simulink library "GenericINSLibrary"  (R2020b)
settings: Solver=VariableStepAuto  StartTime=0.0  StopTime=10.0  RelTol=1e-3
libraries: simulink x44
(part 2 of 6)

== system GenericINSLibrary/Empty Bus Sensor Fusion/GNSS4 ==
  Bus Creator : BusCreator  Inputs=1
  Bus Creator1 : BusCreator  Inputs=3
  Bus Creator2 : BusCreator  Inputs=3
  Bus Creator3 : BusCreator  Inputs=4
  Constant71 : Constant  Value=[0;0;0]  OutDataTypeStr=double
  Constant72 : Constant  OutDataTypeStr=double
  Constant73 : Constant  OutDataTypeStr=double
  Constant74 : Constant  OutDataTypeStr=double
  Constant{75..78} (4 alike) : Constant  Value=0  OutDataTypeStr=double
  Signal Specification : SignalSpecification  OutDataTypeStr=double  Unit=m  Dimensions=3
  Signal Specification{1..3,7} (4 alike) : SignalSpecification  OutDataTypeStr=double  Unit=m  Dimensions=1
  Signal Specification4 : SignalSpecification  OutDataTypeStr=double  Unit=s  Dimensions=1
  Signal Specification5 : SignalSpecification  OutDataTypeStr=double  Unit=rad  Dimensions=1
  Signal Specification6 : SignalSpecification  OutDataTypeStr=double  Unit=rad  Dimensions=1
  busGNSS : Outport
  wires:
  Signal Specification6/1 -> Bus Creator3/3  "longitude"
  Constant72/1 -> Signal Specification1/1
  Signal Specification1/1 -> Bus Creator2/1  "north"
  Constant77/1 -> Signal Specification6/1
  Constant76/1 -> Signal Specification5/1
  Constant71/1 -> Signal Specification/1
  Constant73/1 -> Signal Specification2/1
  Signal Specification7/1 -> Bus Creator3/4  "altitude"
  Constant78/1 -> Signal Specification7/1
  Signal Specification5/1 -> Bus Creator3/2  "latitude"
  Bus Creator2/1 -> Bus Creator1/2  "standardDeviation"
  Bus Creator3/1 -> Bus Creator1/3  "measurement"
  Signal Specification3/1 -> Bus Creator2/3  "down"
  Bus Creator/1 -> Bus Creator1/1  "alignment"
  Constant74/1 -> Signal Specification3/1
  Signal Specification2/1 -> Bus Creator2/2  "east"
  Signal Specification/1 -> Bus Creator/1  "positionBodyToSensor"
  Constant75/1 -> Signal Specification4/1
  Signal Specification4/1 -> Bus Creator3/1  "timestamp"
  Bus Creator1/1 -> busGNSS/1

== system GenericINSLibrary/Empty Bus Sensor Fusion/GNSS5 ==
  Bus Creator : BusCreator  Inputs=1
  Bus Creator1 : BusCreator  Inputs=3
  Bus Creator2 : BusCreator  Inputs=3
  Bus Creator3 : BusCreator  Inputs=4
  Constant71 : Constant  Value=[0;0;0]  OutDataTypeStr=double
  Constant72 : Constant  OutDataTypeStr=double
  Constant73 : Constant  OutDataTypeStr=double
  Constant74 : Constant  OutDataTypeStr=double
  Constant{75..78} (4 alike) : Constant  Value=0  OutDataTypeStr=double
  Signal Specification : SignalSpecification  OutDataTypeStr=double  Unit=m  Dimensions=3
  Signal Specification{1..3,7} (4 alike) : SignalSpecification  OutDataTypeStr=double  Unit=m  Dimensions=1
  Signal Specification4 : SignalSpecification  OutDataTypeStr=double  Unit=s  Dimensions=1
  Signal Specification5 : SignalSpecification  OutDataTypeStr=double  Unit=rad  Dimensions=1
  Signal Specification6 : SignalSpecification  OutDataTypeStr=double  Unit=rad  Dimensions=1
  busGNSS : Outport
  wires:
  Bus Creator1/1 -> busGNSS/1
  Signal Specification4/1 -> Bus Creator3/1  "timestamp"
  Constant75/1 -> Signal Specification4/1
  Signal Specification/1 -> Bus Creator/1  "positionBodyToSensor"
  Signal Specification2/1 -> Bus Creator2/2  "east"
  Constant74/1 -> Signal Specification3/1
  Bus Creator/1 -> Bus Creator1/1  "alignment"
  Signal Specification3/1 -> Bus Creator2/3  "down"
  Bus Creator3/1 -> Bus Creator1/3  "measurement"
  Bus Creator2/1 -> Bus Creator1/2  "standardDeviation"
  Signal Specification5/1 -> Bus Creator3/2  "latitude"
  Constant78/1 -> Signal Specification7/1
  Signal Specification7/1 -> Bus Creator3/4  "altitude"
  Constant73/1 -> Signal Specification2/1
  Constant71/1 -> Signal Specification/1
  Constant76/1 -> Signal Specification5/1
  Constant77/1 -> Signal Specification6/1
  Signal Specification1/1 -> Bus Creator2/1  "north"
  Constant72/1 -> Signal Specification1/1
  Signal Specification6/1 -> Bus Creator3/3  "longitude"

== system GenericINSLibrary/Empty Bus Sensor Fusion/GNSS6 ==
  Bus Creator : BusCreator  Inputs=1
  Bus Creator1 : BusCreator  Inputs=3
  Bus Creator2 : BusCreator  Inputs=3
  Bus Creator3 : BusCreator  Inputs=4
  Constant71 : Constant  Value=[0;0;0]  OutDataTypeStr=double
  Constant72 : Constant  OutDataTypeStr=double
  Constant73 : Constant  OutDataTypeStr=double
  Constant74 : Constant  OutDataTypeStr=double
  Constant{75..78} (4 alike) : Constant  Value=0  OutDataTypeStr=double
  Signal Specification : SignalSpecification  OutDataTypeStr=double  Unit=m  Dimensions=3
  Signal Specification{1..3,7} (4 alike) : SignalSpecification  OutDataTypeStr=double  Unit=m  Dimensions=1
  Signal Specification4 : SignalSpecification  OutDataTypeStr=double  Unit=s  Dimensions=1
  Signal Specification5 : SignalSpecification  OutDataTypeStr=double  Unit=rad  Dimensions=1
  Signal Specification6 : SignalSpecification  OutDataTypeStr=double  Unit=rad  Dimensions=1
  busGNSS : Outport
  wires:
  Signal Specification6/1 -> Bus Creator3/3  "longitude"
  Constant72/1 -> Signal Specification1/1
  Signal Specification1/1 -> Bus Creator2/1  "north"
  Constant77/1 -> Signal Specification6/1
  Constant76/1 -> Signal Specification5/1
  Constant71/1 -> Signal Specification/1
  Constant73/1 -> Signal Specification2/1
  Signal Specification7/1 -> Bus Creator3/4  "altitude"
  Constant78/1 -> Signal Specification7/1
  Signal Specification5/1 -> Bus Creator3/2  "latitude"
  Bus Creator2/1 -> Bus Creator1/2  "standardDeviation"
  Bus Creator3/1 -> Bus Creator1/3  "measurement"
  Signal Specification3/1 -> Bus Creator2/3  "down"
  Bus Creator/1 -> Bus Creator1/1  "alignment"
  Constant74/1 -> Signal Specification3/1
  Signal Specification2/1 -> Bus Creator2/2  "east"
  Signal Specification/1 -> Bus Creator/1  "positionBodyToSensor"
  Constant75/1 -> Signal Specification4/1
  Signal Specification4/1 -> Bus Creator3/1  "timestamp"
  Bus Creator1/1 -> busGNSS/1

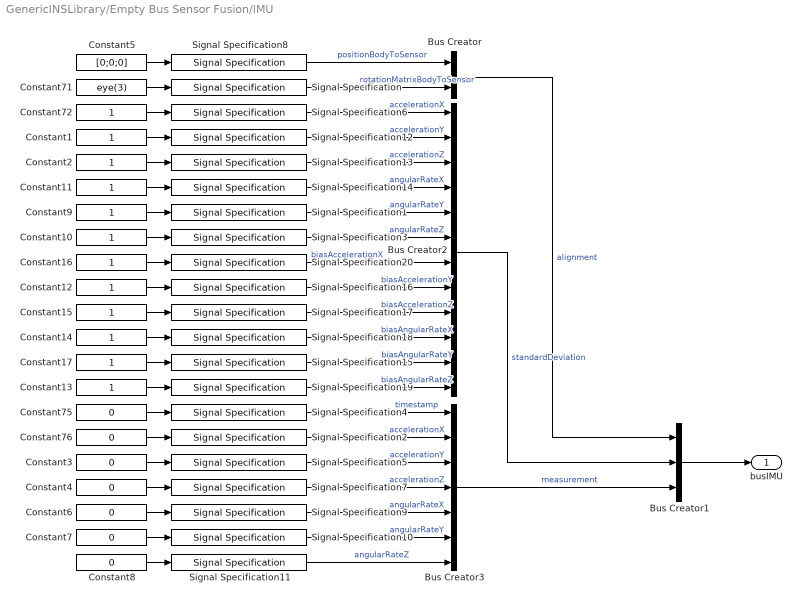
== system GenericINSLibrary/Empty Bus Sensor Fusion/IMU ==
  Bus Creator : BusCreator  Inputs=2
  Bus Creator1 : BusCreator  Inputs=3
  Bus Creator2 : BusCreator  Inputs=12
  Bus Creator3 : BusCreator  Inputs=7
  Constant{1..2,9..17,72} (12 alike) : Constant  OutDataTypeStr=double
  Constant{3..4,6..8,75..76} (7 alike) : Constant  Value=0  OutDataTypeStr=double
  Constant5 : Constant  Value=[0;0;0]  OutDataTypeStr=double
  Constant71 : Constant  Value=eye(3)  OutDataTypeStr=double
  Signal Specification : SignalSpecification  OutDataTypeStr=double  Dimensions=[3 3]
  Signal Specification{1,3,9..11,14..15,18..19} (9 alike) : SignalSpecification  OutDataTypeStr=double  Unit=rad/s  Dimensions=1
  Signal Specification{2,5..7,12..13,16..17,20} (9 alike) : SignalSpecification  OutDataTypeStr=double  Unit=m/s^2  Dimensions=1
  Signal Specification4 : SignalSpecification  OutDataTypeStr=double  Unit=s  Dimensions=1
  Signal Specification8 : SignalSpecification  OutDataTypeStr=double  Unit=m  Dimensions=3
  busIMU : Outport
  wires:
  Constant15/1 -> Signal Specification17/1
  Constant16/1 -> Signal Specification20/1
  Constant12/1 -> Signal Specification16/1
  Signal Specification19/1 -> Bus Creator2/12  "biasAngularRateZ"
  Signal Specification15/1 -> Bus Creator2/11  "biasAngularRateY"
  Signal Specification18/1 -> Bus Creator2/10  "biasAngularRateX"
  Signal Specification17/1 -> Bus Creator2/9  "biasAccelerationZ"
  Signal Specification16/1 -> Bus Creator2/8  "biasAccelerationY"
  Signal Specification20/1 -> Bus Creator2/7  "biasAccelerationX"
  Constant17/1 -> Signal Specification15/1
  Constant14/1 -> Signal Specification18/1
  Constant13/1 -> Signal Specification19/1
  Constant10/1 -> Signal Specification3/1
  Constant11/1 -> Signal Specification14/1
  Constant9/1 -> Signal Specification1/1
  Signal Specification6/1 -> Bus Creator2/1  "accelerationX"
  Signal Specification12/1 -> Bus Creator2/2  "accelerationY"
  Signal Specification13/1 -> Bus Creator2/3  "accelerationZ"
  Signal Specification14/1 -> Bus Creator2/4  "angularRateX"
  Signal Specification1/1 -> Bus Creator2/5  "angularRateY"
  Signal Specification3/1 -> Bus Creator2/6  "angularRateZ"
  Signal Specification11/1 -> Bus Creator3/7  "angularRateZ"
  Signal Specification10/1 -> Bus Creator3/6  "angularRateY"
  Constant8/1 -> Signal Specification11/1
  Constant7/1 -> Signal Specification10/1
  Signal Specification9/1 -> Bus Creator3/5  "angularRateX"
  Constant6/1 -> Signal Specification9/1
  Signal Specification7/1 -> Bus Creator3/4  "accelerationZ"
  Signal Specification5/1 -> Bus Creator3/3  "accelerationY"
  Constant5/1 -> Signal Specification8/1
  Signal Specification8/1 -> Bus Creator/1  "positionBodyToSensor"
  Constant3/1 -> Signal Specification5/1
  Constant1/1 -> Signal Specification12/1
  Signal Specification2/1 -> Bus Creator3/2  "accelerationX"
  Constant72/1 -> Signal Specification6/1
  Constant76/1 -> Signal Specification2/1
  Constant71/1 -> Signal Specification/1
  Bus Creator2/1 -> Bus Creator1/2  "standardDeviation"
  Bus Creator3/1 -> Bus Creator1/3  "measurement"
  Bus Creator/1 -> Bus Creator1/1  "alignment"
  Signal Specification/1 -> Bus Creator/2  "rotationMatrixBodyToSensor"
  Constant75/1 -> Signal Specification4/1
  Signal Specification4/1 -> Bus Creator3/1  "timestamp"
  Bus Creator1/1 -> busIMU/1
  Constant2/1 -> Signal Specification13/1
  Constant4/1 -> Signal Specification7/1

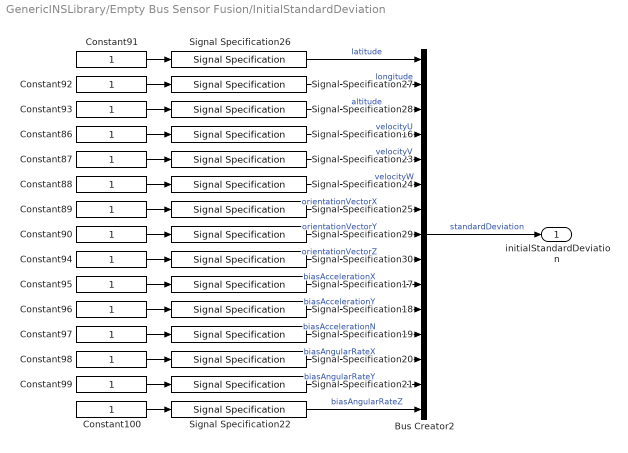
== system GenericINSLibrary/Empty Bus Sensor Fusion/InitialStandardDeviation ==
  Bus Creator2 : BusCreator  Inputs=15
  Constant{86..100} (15 alike) : Constant  OutDataTypeStr=double
  Signal Specification16 : SignalSpecification  OutDataTypeStr=double  Unit=m/s  Dimensions=1
  Signal Specification17 : SignalSpecification  OutDataTypeStr=double  Unit=m/s^2  Dimensions=1
  Signal Specification18 : SignalSpecification  OutDataTypeStr=double  Unit=m/s^2  Dimensions=1
  Signal Specification19 : SignalSpecification  OutDataTypeStr=double  Unit=m/s^2  Dimensions=1
  Signal Specification20 : SignalSpecification  OutDataTypeStr=double  Unit=rad/s  Dimensions=1
  Signal Specification21 : SignalSpecification  OutDataTypeStr=double  Unit=rad/s  Dimensions=1
  Signal Specification22 : SignalSpecification  OutDataTypeStr=double  Unit=rad/s  Dimensions=1
  Signal Specification23 : SignalSpecification  OutDataTypeStr=double  Unit=m/s  Dimensions=1
  Signal Specification24 : SignalSpecification  OutDataTypeStr=double  Unit=m/s  Dimensions=1
  Signal Specification{25..27,29..30} (5 alike) : SignalSpecification  OutDataTypeStr=double  Unit=rad  Dimensions=1
  Signal Specification28 : SignalSpecification  OutDataTypeStr=double  Unit=m  Dimensions=1
  initialStandardDeviation : Outport
  wires:
  Signal Specification29/1 -> Bus Creator2/8  "orientationVectorY"
  Signal Specification18/1 -> Bus Creator2/11  "biasAccelerationY"
  Signal Specification17/1 -> Bus Creator2/10  "biasAccelerationX"
  Signal Specification30/1 -> Bus Creator2/9  "orientationVectorZ"
  Constant97/1 -> Signal Specification19/1
  Constant96/1 -> Signal Specification18/1
  Constant99/1 -> Signal Specification21/1
  Constant98/1 -> Signal Specification20/1
  Bus Creator2/1 -> initialStandardDeviation/1  "standardDeviation"
  Signal Specification20/1 -> Bus Creator2/13  "biasAngularRateX"
  Signal Specification22/1 -> Bus Creator2/15  "biasAngularRateZ"
  Constant100/1 -> Signal Specification22/1
  Signal Specification19/1 -> Bus Creator2/12  "biasAccelerationN"
  Signal Specification28/1 -> Bus Creator2/3  "altitude"
  Constant95/1 -> Signal Specification17/1
  Constant91/1 -> Signal Specification26/1
  Constant92/1 -> Signal Specification27/1
  Constant93/1 -> Signal Specification28/1
  Constant86/1 -> Signal Specification16/1
  Signal Specification24/1 -> Bus Creator2/6  "velocityW"
  Constant87/1 -> Signal Specification23/1
  Signal Specification27/1 -> Bus Creator2/2  "longitude"
  Constant88/1 -> Signal Specification24/1
  Signal Specification26/1 -> Bus Creator2/1  "latitude"
  Signal Specification16/1 -> Bus Creator2/4  "velocityU"
  Constant89/1 -> Signal Specification25/1
  Signal Specification21/1 -> Bus Creator2/14  "biasAngularRateY"
  Constant94/1 -> Signal Specification30/1
  Constant90/1 -> Signal Specification29/1
  Signal Specification23/1 -> Bus Creator2/5  "velocityV"
  Signal Specification25/1 -> Bus Creator2/7  "orientationVectorX"

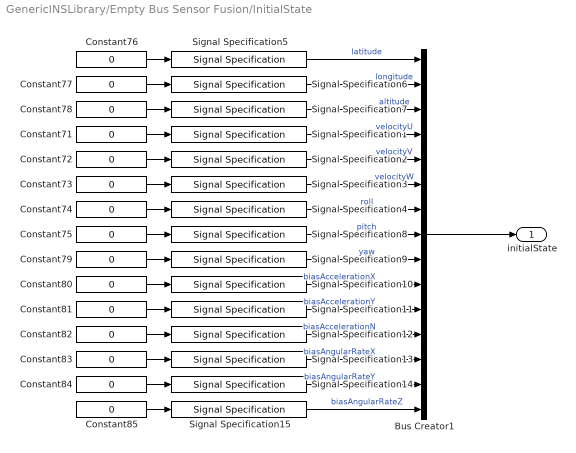
== system GenericINSLibrary/Empty Bus Sensor Fusion/InitialState ==
  Bus Creator1 : BusCreator  Inputs=15
  Constant{71..85} (15 alike) : Constant  Value=0  OutDataTypeStr=double
  Signal Specification1 : SignalSpecification  OutDataTypeStr=double  Unit=m/s  Dimensions=1
  Signal Specification10 : SignalSpecification  OutDataTypeStr=double  Unit=m/s^2  Dimensions=1
  Signal Specification11 : SignalSpecification  OutDataTypeStr=double  Unit=m/s^2  Dimensions=1
  Signal Specification12 : SignalSpecification  OutDataTypeStr=double  Unit=m/s^2  Dimensions=1
  Signal Specification13 : SignalSpecification  OutDataTypeStr=double  Unit=rad/s  Dimensions=1
  Signal Specification14 : SignalSpecification  OutDataTypeStr=double  Unit=rad/s  Dimensions=1
  Signal Specification15 : SignalSpecification  OutDataTypeStr=double  Unit=rad/s  Dimensions=1
  Signal Specification2 : SignalSpecification  OutDataTypeStr=double  Unit=m/s  Dimensions=1
  Signal Specification3 : SignalSpecification  OutDataTypeStr=double  Unit=m/s  Dimensions=1
  Signal Specification{4..6,8..9} (5 alike) : SignalSpecification  OutDataTypeStr=double  Unit=rad  Dimensions=1
  Signal Specification7 : SignalSpecification  OutDataTypeStr=double  Unit=m  Dimensions=1
  initialState : Outport
  wires:
  Signal Specification10/1 -> Bus Creator1/10  "biasAccelerationX"
  Constant74/1 -> Signal Specification4/1
  Constant78/1 -> Signal Specification7/1
  Bus Creator1/1 -> initialState/1
  Constant76/1 -> Signal Specification5/1
  Constant77/1 -> Signal Specification6/1
  Signal Specification14/1 -> Bus Creator1/14  "biasAngularRateY"
  Constant72/1 -> Signal Specification2/1
  Constant85/1 -> Signal Specification15/1
  Signal Specification12/1 -> Bus Creator1/12  "biasAccelerationN"
  Signal Specification15/1 -> Bus Creator1/15  "biasAngularRateZ"
  Signal Specification1/1 -> Bus Creator1/4  "velocityU"
  Signal Specification3/1 -> Bus Creator1/6  "velocityW"
  Signal Specification8/1 -> Bus Creator1/8  "pitch"
  Constant83/1 -> Signal Specification13/1
  Signal Specification7/1 -> Bus Creator1/3  "altitude"
  Signal Specification5/1 -> Bus Creator1/1  "latitude"
  Constant75/1 -> Signal Specification8/1
  Constant71/1 -> Signal Specification1/1
  Constant84/1 -> Signal Specification14/1
  Signal Specification13/1 -> Bus Creator1/13  "biasAngularRateX"
  Signal Specification2/1 -> Bus Creator1/5  "velocityV"
  Constant81/1 -> Signal Specification11/1
  Constant80/1 -> Signal Specification10/1
  Signal Specification9/1 -> Bus Creator1/9  "yaw"
  Constant79/1 -> Signal Specification9/1
  Constant82/1 -> Signal Specification12/1
  Constant73/1 -> Signal Specification3/1
  Signal Specification6/1 -> Bus Creator1/2  "longitude"
  Signal Specification4/1 -> Bus Creator1/7  "roll"
  Signal Specification11/1 -> Bus Creator1/11  "biasAccelerationY"

== system GenericINSLibrary/Empty Bus Sensor Fusion/SOG1 ==
  Bus Creator : BusCreator  Inputs=1
  Bus Creator1 : BusCreator  Inputs=3
  Bus Creator2 : BusCreator  Inputs=1
  Bus Creator3 : BusCreator  Inputs=2
  Constant71 : Constant  Value=[0;0;0]  OutDataTypeStr=double
  Constant72 : Constant  OutDataTypeStr=double
  Constant75 : Constant  Value=0  OutDataTypeStr=double
  Constant76 : Constant  Value=0  OutDataTypeStr=double
  Signal Specification : SignalSpecification  OutDataTypeStr=double  Unit=m  Dimensions=3
  Signal Specification1 : SignalSpecification  OutDataTypeStr=double  Unit=m/s  Dimensions=1
  Signal Specification2 : SignalSpecification  OutDataTypeStr=double  Unit=m/s  Dimensions=1
  Signal Specification4 : SignalSpecification  OutDataTypeStr=double  Unit=s  Dimensions=1
  busSOG : Outport
  wires:
  Signal Specification2/1 -> Bus Creator3/2  "speedOverGround"
  Constant72/1 -> Signal Specification1/1
  Signal Specification1/1 -> Bus Creator2/1  "speedOverGround"
  Constant76/1 -> Signal Specification2/1
  Constant71/1 -> Signal Specification/1
  Bus Creator2/1 -> Bus Creator1/2  "standardDeviation"
  Bus Creator3/1 -> Bus Creator1/3  "measurement"
  Bus Creator/1 -> Bus Creator1/1  "alignment"
  Signal Specification/1 -> Bus Creator/1  "positionBodyToSensor"
  Constant75/1 -> Signal Specification4/1
  Signal Specification4/1 -> Bus Creator3/1  "timestamp"
  Bus Creator1/1 -> busSOG/1

== system GenericINSLibrary/Empty Bus Sensor Fusion/SOG2 ==
  Bus Creator : BusCreator  Inputs=1
  Bus Creator1 : BusCreator  Inputs=3
  Bus Creator2 : BusCreator  Inputs=1
  Bus Creator3 : BusCreator  Inputs=2
  Constant71 : Constant  Value=[0;0;0]  OutDataTypeStr=double
  Constant72 : Constant  OutDataTypeStr=double
  Constant75 : Constant  Value=0  OutDataTypeStr=double
  Constant76 : Constant  Value=0  OutDataTypeStr=double
  Signal Specification : SignalSpecification  OutDataTypeStr=double  Unit=m  Dimensions=3
  Signal Specification1 : SignalSpecification  OutDataTypeStr=double  Unit=m/s  Dimensions=1
  Signal Specification2 : SignalSpecification  OutDataTypeStr=double  Unit=m/s  Dimensions=1
  Signal Specification4 : SignalSpecification  OutDataTypeStr=double  Unit=s  Dimensions=1
  busSOG : Outport
  wires:
  Bus Creator1/1 -> busSOG/1
  Signal Specification4/1 -> Bus Creator3/1  "timestamp"
  Constant75/1 -> Signal Specification4/1
  Signal Specification/1 -> Bus Creator/1  "positionBodyToSensor"
  Bus Creator/1 -> Bus Creator1/1  "alignment"
  Bus Creator3/1 -> Bus Creator1/3  "measurement"
  Bus Creator2/1 -> Bus Creator1/2  "standardDeviation"
  Constant71/1 -> Signal Specification/1
  Constant76/1 -> Signal Specification2/1
  Signal Specification1/1 -> Bus Creator2/1  "speedOverGround"
  Constant72/1 -> Signal Specification1/1
  Signal Specification2/1 -> Bus Creator3/2  "speedOverGround"

== system GenericINSLibrary/Empty Bus Sensor Fusion/SOG3 ==
  Bus Creator : BusCreator  Inputs=1
  Bus Creator1 : BusCreator  Inputs=3
  Bus Creator2 : BusCreator  Inputs=1
  Bus Creator3 : BusCreator  Inputs=2
  Constant71 : Constant  Value=[0;0;0]  OutDataTypeStr=double
  Constant72 : Constant  OutDataTypeStr=double
  Constant75 : Constant  Value=0  OutDataTypeStr=double
  Constant76 : Constant  Value=0  OutDataTypeStr=double
  Signal Specification : SignalSpecification  OutDataTypeStr=double  Unit=m  Dimensions=3
  Signal Specification1 : SignalSpecification  OutDataTypeStr=double  Unit=m/s  Dimensions=1
  Signal Specification2 : SignalSpecification  OutDataTypeStr=double  Unit=m/s  Dimensions=1
  Signal Specification4 : SignalSpecification  OutDataTypeStr=double  Unit=s  Dimensions=1
  busSOG : Outport
  wires:
  Signal Specification2/1 -> Bus Creator3/2  "speedOverGround"
  Constant72/1 -> Signal Specification1/1
  Signal Specification1/1 -> Bus Creator2/1  "speedOverGround"
  Constant76/1 -> Signal Specification2/1
  Constant71/1 -> Signal Specification/1
  Bus Creator2/1 -> Bus Creator1/2  "standardDeviation"
  Bus Creator3/1 -> Bus Creator1/3  "measurement"
  Bus Creator/1 -> Bus Creator1/1  "alignment"
  Signal Specification/1 -> Bus Creator/1  "positionBodyToSensor"
  Constant75/1 -> Signal Specification4/1
  Signal Specification4/1 -> Bus Creator3/1  "timestamp"
  Bus Creator1/1 -> busSOG/1

== system GenericINSLibrary/Empty Bus Sensor Fusion/SOG4 ==
  Bus Creator : BusCreator  Inputs=1
  Bus Creator1 : BusCreator  Inputs=3
  Bus Creator2 : BusCreator  Inputs=1
  Bus Creator3 : BusCreator  Inputs=2
  Constant71 : Constant  Value=[0;0;0]  OutDataTypeStr=double
  Constant72 : Constant  OutDataTypeStr=double
  Constant75 : Constant  Value=0  OutDataTypeStr=double
  Constant76 : Constant  Value=0  OutDataTypeStr=double
  Signal Specification : SignalSpecification  OutDataTypeStr=double  Unit=m  Dimensions=3
  Signal Specification1 : SignalSpecification  OutDataTypeStr=double  Unit=m/s  Dimensions=1
  Signal Specification2 : SignalSpecification  OutDataTypeStr=double  Unit=m/s  Dimensions=1
  Signal Specification4 : SignalSpecification  OutDataTypeStr=double  Unit=s  Dimensions=1
  busSOG : Outport
  wires:
  Bus Creator1/1 -> busSOG/1
  Signal Specification4/1 -> Bus Creator3/1  "timestamp"
  Constant75/1 -> Signal Specification4/1
  Signal Specification/1 -> Bus Creator/1  "positionBodyToSensor"
  Bus Creator/1 -> Bus Creator1/1  "alignment"
  Bus Creator3/1 -> Bus Creator1/3  "measurement"
  Bus Creator2/1 -> Bus Creator1/2  "standardDeviation"
  Constant71/1 -> Signal Specification/1
  Constant76/1 -> Signal Specification2/1
  Signal Specification1/1 -> Bus Creator2/1  "speedOverGround"
  Constant72/1 -> Signal Specification1/1
  Signal Specification2/1 -> Bus Creator3/2  "speedOverGround"

== system GenericINSLibrary/Empty Bus Sensor Fusion/SOG5 ==
  Bus Creator : BusCreator  Inputs=1
  Bus Creator1 : BusCreator  Inputs=3
  Bus Creator2 : BusCreator  Inputs=1
  Bus Creator3 : BusCreator  Inputs=2
  Constant71 : Constant  Value=[0;0;0]  OutDataTypeStr=double
  Constant72 : Constant  OutDataTypeStr=double
  Constant75 : Constant  Value=0  OutDataTypeStr=double
  Constant76 : Constant  Value=0  OutDataTypeStr=double
  Signal Specification : SignalSpecification  OutDataTypeStr=double  Unit=m  Dimensions=3
  Signal Specification1 : SignalSpecification  OutDataTypeStr=double  Unit=m/s  Dimensions=1
  Signal Specification2 : SignalSpecification  OutDataTypeStr=double  Unit=m/s  Dimensions=1
  Signal Specification4 : SignalSpecification  OutDataTypeStr=double  Unit=s  Dimensions=1
  busSOG : Outport
  wires:
  Signal Specification2/1 -> Bus Creator3/2  "speedOverGround"
  Constant72/1 -> Signal Specification1/1
  Signal Specification1/1 -> Bus Creator2/1  "speedOverGround"
  Constant76/1 -> Signal Specification2/1
  Constant71/1 -> Signal Specification/1
  Bus Creator2/1 -> Bus Creator1/2  "standardDeviation"
  Bus Creator3/1 -> Bus Creator1/3  "measurement"
  Bus Creator/1 -> Bus Creator1/1  "alignment"
  Signal Specification/1 -> Bus Creator/1  "positionBodyToSensor"
  Constant75/1 -> Signal Specification4/1
  Signal Specification4/1 -> Bus Creator3/1  "timestamp"
  Bus Creator1/1 -> busSOG/1

== system GenericINSLibrary/Empty Bus Sensor Fusion/SOG6 ==
  Bus Creator : BusCreator  Inputs=1
  Bus Creator1 : BusCreator  Inputs=3
  Bus Creator2 : BusCreator  Inputs=1
  Bus Creator3 : BusCreator  Inputs=2
  Constant71 : Constant  Value=[0;0;0]  OutDataTypeStr=double
  Constant72 : Constant  OutDataTypeStr=double
  Constant75 : Constant  Value=0  OutDataTypeStr=double
  Constant76 : Constant  Value=0  OutDataTypeStr=double
  Signal Specification : SignalSpecification  OutDataTypeStr=double  Unit=m  Dimensions=3
  Signal Specification1 : SignalSpecification  OutDataTypeStr=double  Unit=m/s  Dimensions=1
  Signal Specification2 : SignalSpecification  OutDataTypeStr=double  Unit=m/s  Dimensions=1
  Signal Specification4 : SignalSpecification  OutDataTypeStr=double  Unit=s  Dimensions=1
  busSOG : Outport
  wires:
  Bus Creator1/1 -> busSOG/1
  Signal Specification4/1 -> Bus Creator3/1  "timestamp"
  Constant75/1 -> Signal Specification4/1
  Signal Specification/1 -> Bus Creator/1  "positionBodyToSensor"
  Bus Creator/1 -> Bus Creator1/1  "alignment"
  Bus Creator3/1 -> Bus Creator1/3  "measurement"
  Bus Creator2/1 -> Bus Creator1/2  "standardDeviation"
  Constant71/1 -> Signal Specification/1
  Constant76/1 -> Signal Specification2/1
  Signal Specification1/1 -> Bus Creator2/1  "speedOverGround"
  Constant72/1 -> Signal Specification1/1
  Signal Specification2/1 -> Bus Creator3/2  "speedOverGround"

== system GenericINSLibrary/Empty Bus Sensor Fusion/VelocityXY1 ==
  Bus Creator : BusCreator  Inputs=2
  Bus Creator1 : BusCreator  Inputs=3
  Bus Creator2 : BusCreator  Inputs=2
  Bus Creator3 : BusCreator  Inputs=3
  Constant1 : Constant  OutDataTypeStr=double
  Constant3 : Constant  Value=0  OutDataTypeStr=double
  Constant5 : Constant  Value=[0;0;0]  OutDataTypeStr=double
  Constant71 : Constant  Value=eye(3)  OutDataTypeStr=double
  Constant72 : Constant  OutDataTypeStr=double
  Constant75 : Constant  Value=0  OutDataTypeStr=double
  Constant76 : Constant  Value=0  OutDataTypeStr=double
  Signal Specification : SignalSpecification  OutDataTypeStr=double  Dimensions=[3 3]
  Signal Specification{1..3,5} (4 alike) : SignalSpecification  OutDataTypeStr=double  Unit=m/s  Dimensions=1
  Signal Specification4 : SignalSpecification  OutDataTypeStr=double  Unit=s  Dimensions=1
  Signal Specification8 : SignalSpecification  OutDataTypeStr=double  Unit=m  Dimensions=3
  busVelocityXY : Outport
  wires:
  Constant5/1 -> Signal Specification8/1
  Signal Specification8/1 -> Bus Creator/1  "positionBodyToSensor"
  Constant3/1 -> Signal Specification5/1
  Signal Specification5/1 -> Bus Creator3/3  "velocityY"
  Signal Specification3/1 -> Bus Creator2/2  "velocityY"
  Constant1/1 -> Signal Specification3/1
  Signal Specification2/1 -> Bus Creator3/2  "velocityX"
  Constant72/1 -> Signal Specification1/1
  Signal Specification1/1 -> Bus Creator2/1  "velocityX"
  Constant76/1 -> Signal Specification2/1
  Constant71/1 -> Signal Specification/1
  Bus Creator2/1 -> Bus Creator1/2  "standardDeviation"
  Bus Creator3/1 -> Bus Creator1/3  "measurement"
  Bus Creator/1 -> Bus Creator1/1  "alignment"
  Signal Specification/1 -> Bus Creator/2  "rotationMatrixBodyToSensor"
  Constant75/1 -> Signal Specification4/1
  Signal Specification4/1 -> Bus Creator3/1  "timestamp"
  Bus Creator1/1 -> busVelocityXY/1

== system GenericINSLibrary/Empty Bus Sensor Fusion/VelocityXY2 ==
  Bus Creator : BusCreator  Inputs=2
  Bus Creator1 : BusCreator  Inputs=3
  Bus Creator2 : BusCreator  Inputs=2
  Bus Creator3 : BusCreator  Inputs=3
  Constant1 : Constant  OutDataTypeStr=double
  Constant3 : Constant  Value=0  OutDataTypeStr=double
  Constant5 : Constant  Value=[0;0;0]  OutDataTypeStr=double
  Constant71 : Constant  Value=eye(3)  OutDataTypeStr=double
  Constant72 : Constant  OutDataTypeStr=double
  Constant75 : Constant  Value=0  OutDataTypeStr=double
  Constant76 : Constant  Value=0  OutDataTypeStr=double
  Signal Specification : SignalSpecification  OutDataTypeStr=double  Dimensions=[3 3]
  Signal Specification{1..3,5} (4 alike) : SignalSpecification  OutDataTypeStr=double  Unit=m/s  Dimensions=1
  Signal Specification4 : SignalSpecification  OutDataTypeStr=double  Unit=s  Dimensions=1
  Signal Specification8 : SignalSpecification  OutDataTypeStr=double  Unit=m  Dimensions=3
  busVelocityXY : Outport
  wires:
  Bus Creator1/1 -> busVelocityXY/1
  Signal Specification4/1 -> Bus Creator3/1  "timestamp"
  Constant75/1 -> Signal Specification4/1
  Signal Specification/1 -> Bus Creator/2  "rotationMatrixBodyToSensor"
  Bus Creator/1 -> Bus Creator1/1  "alignment"
  Bus Creator3/1 -> Bus Creator1/3  "measurement"
  Bus Creator2/1 -> Bus Creator1/2  "standardDeviation"
  Constant71/1 -> Signal Specification/1
  Constant76/1 -> Signal Specification2/1
  Signal Specification1/1 -> Bus Creator2/1  "velocityX"
  Constant72/1 -> Signal Specification1/1
  Signal Specification2/1 -> Bus Creator3/2  "velocityX"
  Constant1/1 -> Signal Specification3/1
  Signal Specification3/1 -> Bus Creator2/2  "velocityY"
  Signal Specification5/1 -> Bus Creator3/3  "velocityY"
  Constant3/1 -> Signal Specification5/1
  Signal Specification8/1 -> Bus Creator/1  "positionBodyToSensor"
  Constant5/1 -> Signal Specification8/1

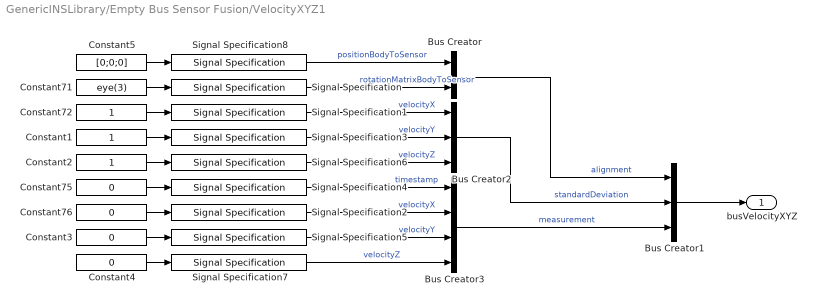
== system GenericINSLibrary/Empty Bus Sensor Fusion/VelocityXYZ1 ==
  Bus Creator : BusCreator  Inputs=2
  Bus Creator1 : BusCreator  Inputs=3
  Bus Creator2 : BusCreator  Inputs=3
  Bus Creator3 : BusCreator  Inputs=4
  Constant1 : Constant  OutDataTypeStr=double
  Constant2 : Constant  OutDataTypeStr=double
  Constant{3..4,75..76} (4 alike) : Constant  Value=0  OutDataTypeStr=double
  Constant5 : Constant  Value=[0;0;0]  OutDataTypeStr=double
  Constant71 : Constant  Value=eye(3)  OutDataTypeStr=double
  Constant72 : Constant  OutDataTypeStr=double
  Signal Specification : SignalSpecification  OutDataTypeStr=double  Dimensions=[3 3]
  Signal Specification{1..3,5..7} (6 alike) : SignalSpecification  OutDataTypeStr=double  Unit=m/s  Dimensions=1
  Signal Specification4 : SignalSpecification  OutDataTypeStr=double  Unit=s  Dimensions=1
  Signal Specification8 : SignalSpecification  OutDataTypeStr=double  Unit=m  Dimensions=3
  busVelocityXYZ : Outport
  wires:
  Signal Specification7/1 -> Bus Creator3/4  "velocityZ"
  Constant4/1 -> Signal Specification7/1
  Signal Specification6/1 -> Bus Creator2/3  "velocityZ"
  Constant2/1 -> Signal Specification6/1
  Bus Creator1/1 -> busVelocityXYZ/1
  Signal Specification4/1 -> Bus Creator3/1  "timestamp"
  Constant75/1 -> Signal Specification4/1
  Signal Specification/1 -> Bus Creator/2  "rotationMatrixBodyToSensor"
  Bus Creator/1 -> Bus Creator1/1  "alignment"
  Bus Creator3/1 -> Bus Creator1/3  "measurement"
  Bus Creator2/1 -> Bus Creator1/2  "standardDeviation"
  Constant71/1 -> Signal Specification/1
  Constant76/1 -> Signal Specification2/1
  Signal Specification1/1 -> Bus Creator2/1  "velocityX"
  Constant72/1 -> Signal Specification1/1
  Signal Specification2/1 -> Bus Creator3/2  "velocityX"
  Constant1/1 -> Signal Specification3/1
  Signal Specification3/1 -> Bus Creator2/2  "velocityY"
  Signal Specification5/1 -> Bus Creator3/3  "velocityY"
  Constant3/1 -> Signal Specification5/1
  Signal Specification8/1 -> Bus Creator/1  "positionBodyToSensor"
  Constant5/1 -> Signal Specification8/1

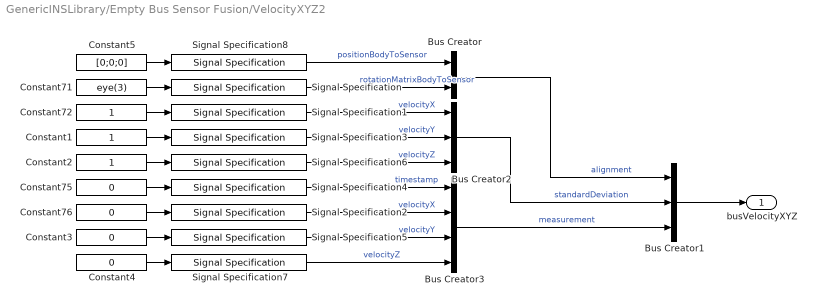
== system GenericINSLibrary/Empty Bus Sensor Fusion/VelocityXYZ2 ==
  Bus Creator : BusCreator  Inputs=2
  Bus Creator1 : BusCreator  Inputs=3
  Bus Creator2 : BusCreator  Inputs=3
  Bus Creator3 : BusCreator  Inputs=4
  Constant1 : Constant  OutDataTypeStr=double
  Constant2 : Constant  OutDataTypeStr=double
  Constant{3..4,75..76} (4 alike) : Constant  Value=0  OutDataTypeStr=double
  Constant5 : Constant  Value=[0;0;0]  OutDataTypeStr=double
  Constant71 : Constant  Value=eye(3)  OutDataTypeStr=double
  Constant72 : Constant  OutDataTypeStr=double
  Signal Specification : SignalSpecification  OutDataTypeStr=double  Dimensions=[3 3]
  Signal Specification{1..3,5..7} (6 alike) : SignalSpecification  OutDataTypeStr=double  Unit=m/s  Dimensions=1
  Signal Specification4 : SignalSpecification  OutDataTypeStr=double  Unit=s  Dimensions=1
  Signal Specification8 : SignalSpecification  OutDataTypeStr=double  Unit=m  Dimensions=3
  busVelocityXYZ : Outport
  wires:
  Constant5/1 -> Signal Specification8/1
  Signal Specification8/1 -> Bus Creator/1  "positionBodyToSensor"
  Constant3/1 -> Signal Specification5/1
  Signal Specification5/1 -> Bus Creator3/3  "velocityY"
  Signal Specification3/1 -> Bus Creator2/2  "velocityY"
  Constant1/1 -> Signal Specification3/1
  Signal Specification2/1 -> Bus Creator3/2  "velocityX"
  Constant72/1 -> Signal Specification1/1
  Signal Specification1/1 -> Bus Creator2/1  "velocityX"
  Constant76/1 -> Signal Specification2/1
  Constant71/1 -> Signal Specification/1
  Bus Creator2/1 -> Bus Creator1/2  "standardDeviation"
  Bus Creator3/1 -> Bus Creator1/3  "measurement"
  Bus Creator/1 -> Bus Creator1/1  "alignment"
  Signal Specification/1 -> Bus Creator/2  "rotationMatrixBodyToSensor"
  Constant75/1 -> Signal Specification4/1
  Signal Specification4/1 -> Bus Creator3/1  "timestamp"
  Bus Creator1/1 -> busVelocityXYZ/1
  Constant2/1 -> Signal Specification6/1
  Signal Specification6/1 -> Bus Creator2/3  "velocityZ"
  Constant4/1 -> Signal Specification7/1
  Signal Specification7/1 -> Bus Creator3/4  "velocityZ"

== system GenericINSLibrary/Empty Bus Sensor Fusion No Bias Estimation/AHRS1 ==
  Bus Creator : BusCreator  Inputs=1
  Bus Creator1 : BusCreator  Inputs=3
  Bus Creator2 : BusCreator  Inputs=3
  Bus Creator3 : BusCreator  Inputs=4
  Constant1 : Constant  OutDataTypeStr=double
  Constant2 : Constant  OutDataTypeStr=double
  Constant{3..4,75..76} (4 alike) : Constant  Value=0  OutDataTypeStr=double
  Constant71 : Constant  Value=eye(3)  OutDataTypeStr=double
  Constant72 : Constant  OutDataTypeStr=double
  Signal Specification : SignalSpecification  OutDataTypeStr=double  Dimensions=[3 3]
  Signal Specification{1..3,5..7} (6 alike) : SignalSpecification  OutDataTypeStr=double  Unit=rad  Dimensions=1
  Signal Specification4 : SignalSpecification  OutDataTypeStr=double  Unit=s  Dimensions=1
  busAHRS : Outport
  wires:
  Bus Creator1/1 -> busAHRS/1
  Signal Specification4/1 -> Bus Creator3/1  "timestamp"
  Constant75/1 -> Signal Specification4/1
  Signal Specification/1 -> Bus Creator/1  "rotationMatrixBodyToSensor"
  Bus Creator/1 -> Bus Creator1/1  "alignment"
  Bus Creator3/1 -> Bus Creator1/3  "measurement"
  Bus Creator2/1 -> Bus Creator1/2  "standardDeviation"
  Constant71/1 -> Signal Specification/1
  Constant76/1 -> Signal Specification2/1
  Signal Specification1/1 -> Bus Creator2/1  "roll"
  Constant72/1 -> Signal Specification1/1
  Signal Specification2/1 -> Bus Creator3/2  "roll"
  Constant1/1 -> Signal Specification3/1
  Constant2/1 -> Signal Specification5/1
  Signal Specification3/1 -> Bus Creator2/2  "pitch"
  Signal Specification5/1 -> Bus Creator2/3  "yaw"
  Signal Specification6/1 -> Bus Creator3/3  "pitch"
  Signal Specification7/1 -> Bus Creator3/4  "yaw"
  Constant3/1 -> Signal Specification6/1
  Constant4/1 -> Signal Specification7/1

== system GenericINSLibrary/Empty Bus Sensor Fusion No Bias Estimation/AHRS2 ==
  Bus Creator : BusCreator  Inputs=1
  Bus Creator1 : BusCreator  Inputs=3
  Bus Creator2 : BusCreator  Inputs=3
  Bus Creator3 : BusCreator  Inputs=4
  Constant1 : Constant  OutDataTypeStr=double
  Constant2 : Constant  OutDataTypeStr=double
  Constant{3..4,75..76} (4 alike) : Constant  Value=0  OutDataTypeStr=double
  Constant71 : Constant  Value=eye(3)  OutDataTypeStr=double
  Constant72 : Constant  OutDataTypeStr=double
  Signal Specification : SignalSpecification  OutDataTypeStr=double  Dimensions=[3 3]
  Signal Specification{1..3,5..7} (6 alike) : SignalSpecification  OutDataTypeStr=double  Unit=rad  Dimensions=1
  Signal Specification4 : SignalSpecification  OutDataTypeStr=double  Unit=s  Dimensions=1
  busAHRS : Outport
  wires:
  Constant4/1 -> Signal Specification7/1
  Constant3/1 -> Signal Specification6/1
  Signal Specification7/1 -> Bus Creator3/4  "yaw"
  Signal Specification6/1 -> Bus Creator3/3  "pitch"
  Signal Specification5/1 -> Bus Creator2/3  "yaw"
  Signal Specification3/1 -> Bus Creator2/2  "pitch"
  Constant2/1 -> Signal Specification5/1
  Constant1/1 -> Signal Specification3/1
  Signal Specification2/1 -> Bus Creator3/2  "roll"
  Constant72/1 -> Signal Specification1/1
  Signal Specification1/1 -> Bus Creator2/1  "roll"
  Constant76/1 -> Signal Specification2/1
  Constant71/1 -> Signal Specification/1
  Bus Creator2/1 -> Bus Creator1/2  "standardDeviation"
  Bus Creator3/1 -> Bus Creator1/3  "measurement"
  Bus Creator/1 -> Bus Creator1/1  "alignment"
  Signal Specification/1 -> Bus Creator/1  "rotationMatrixBodyToSensor"
  Constant75/1 -> Signal Specification4/1
  Signal Specification4/1 -> Bus Creator3/1  "timestamp"
  Bus Creator1/1 -> busAHRS/1

== system GenericINSLibrary/Empty Bus Sensor Fusion No Bias Estimation/Compass1 ==
  Bus Creator : BusCreator  Inputs=1
  Bus Creator1 : BusCreator  Inputs=3
  Bus Creator2 : BusCreator  Inputs=1
  Bus Creator3 : BusCreator  Inputs=2
  Constant71 : Constant  Value=eye(3)  OutDataTypeStr=double
  Constant72 : Constant  OutDataTypeStr=double
  Constant75 : Constant  Value=0  OutDataTypeStr=double
  Constant76 : Constant  Value=0  OutDataTypeStr=double
  Signal Specification : SignalSpecification  OutDataTypeStr=double  Dimensions=[3 3]
  Signal Specification1 : SignalSpecification  OutDataTypeStr=double  Unit=rad  Dimensions=1
  Signal Specification2 : SignalSpecification  OutDataTypeStr=double  Unit=rad  Dimensions=1
  Signal Specification4 : SignalSpecification  OutDataTypeStr=double  Unit=s  Dimensions=1
  busCompass : Outport
  wires:
  Bus Creator1/1 -> busCompass/1
  Signal Specification4/1 -> Bus Creator3/1  "timestamp"
  Constant75/1 -> Signal Specification4/1
  Signal Specification/1 -> Bus Creator/1  "rotationMatrixBodyToSensor"
  Bus Creator/1 -> Bus Creator1/1  "alignment"
  Bus Creator3/1 -> Bus Creator1/3  "measurement"
  Bus Creator2/1 -> Bus Creator1/2  "standardDeviation"
  Constant71/1 -> Signal Specification/1
  Constant76/1 -> Signal Specification2/1
  Signal Specification1/1 -> Bus Creator2/1  "yaw"
  Constant72/1 -> Signal Specification1/1
  Signal Specification2/1 -> Bus Creator3/2  "yaw"

== system GenericINSLibrary/Empty Bus Sensor Fusion No Bias Estimation/Compass2 ==
  Bus Creator : BusCreator  Inputs=1
  Bus Creator1 : BusCreator  Inputs=3
  Bus Creator2 : BusCreator  Inputs=1
  Bus Creator3 : BusCreator  Inputs=2
  Constant71 : Constant  Value=eye(3)  OutDataTypeStr=double
  Constant72 : Constant  OutDataTypeStr=double
  Constant75 : Constant  Value=0  OutDataTypeStr=double
  Constant76 : Constant  Value=0  OutDataTypeStr=double
  Signal Specification : SignalSpecification  OutDataTypeStr=double  Dimensions=[3 3]
  Signal Specification1 : SignalSpecification  OutDataTypeStr=double  Unit=rad  Dimensions=1
  Signal Specification2 : SignalSpecification  OutDataTypeStr=double  Unit=rad  Dimensions=1
  Signal Specification4 : SignalSpecification  OutDataTypeStr=double  Unit=s  Dimensions=1
  busCompass : Outport
  wires:
  Signal Specification2/1 -> Bus Creator3/2  "yaw"
  Constant72/1 -> Signal Specification1/1
  Signal Specification1/1 -> Bus Creator2/1  "yaw"
  Constant76/1 -> Signal Specification2/1
  Constant71/1 -> Signal Specification/1
  Bus Creator2/1 -> Bus Creator1/2  "standardDeviation"
  Bus Creator3/1 -> Bus Creator1/3  "measurement"
  Bus Creator/1 -> Bus Creator1/1  "alignment"
  Signal Specification/1 -> Bus Creator/1  "rotationMatrixBodyToSensor"
  Constant75/1 -> Signal Specification4/1
  Signal Specification4/1 -> Bus Creator3/1  "timestamp"
  Bus Creator1/1 -> busCompass/1

== system GenericINSLibrary/Empty Bus Sensor Fusion No Bias Estimation/GNSS1 ==
  Bus Creator : BusCreator  Inputs=1
  Bus Creator1 : BusCreator  Inputs=3
  Bus Creator2 : BusCreator  Inputs=3
  Bus Creator3 : BusCreator  Inputs=4
  Constant71 : Constant  Value=[0;0;0]  OutDataTypeStr=double
  Constant72 : Constant  OutDataTypeStr=double
  Constant73 : Constant  OutDataTypeStr=double
  Constant74 : Constant  OutDataTypeStr=double
  Constant{75..78} (4 alike) : Constant  Value=0  OutDataTypeStr=double
  Signal Specification : SignalSpecification  OutDataTypeStr=double  Unit=m  Dimensions=3
  Signal Specification{1..3,7} (4 alike) : SignalSpecification  OutDataTypeStr=double  Unit=m  Dimensions=1
  Signal Specification4 : SignalSpecification  OutDataTypeStr=double  Unit=s  Dimensions=1
  Signal Specification5 : SignalSpecification  OutDataTypeStr=double  Unit=rad  Dimensions=1
  Signal Specification6 : SignalSpecification  OutDataTypeStr=double  Unit=rad  Dimensions=1
  busGNSS : Outport
  wires:
  Signal Specification6/1 -> Bus Creator3/3  "longitude"
  Constant72/1 -> Signal Specification1/1
  Signal Specification1/1 -> Bus Creator2/1  "north"
  Constant77/1 -> Signal Specification6/1
  Constant76/1 -> Signal Specification5/1
  Constant71/1 -> Signal Specification/1
  Constant73/1 -> Signal Specification2/1
  Signal Specification7/1 -> Bus Creator3/4  "altitude"
  Constant78/1 -> Signal Specification7/1
  Signal Specification5/1 -> Bus Creator3/2  "latitude"
  Bus Creator2/1 -> Bus Creator1/2  "standardDeviation"
  Bus Creator3/1 -> Bus Creator1/3  "measurement"
  Signal Specification3/1 -> Bus Creator2/3  "down"
  Bus Creator/1 -> Bus Creator1/1  "alignment"
  Constant74/1 -> Signal Specification3/1
  Signal Specification2/1 -> Bus Creator2/2  "east"
  Signal Specification/1 -> Bus Creator/1  "positionBodyToSensor"
  Constant75/1 -> Signal Specification4/1
  Signal Specification4/1 -> Bus Creator3/1  "timestamp"
  Bus Creator1/1 -> busGNSS/1

== system GenericINSLibrary/Empty Bus Sensor Fusion No Bias Estimation/GNSS2 ==
  Bus Creator : BusCreator  Inputs=1
  Bus Creator1 : BusCreator  Inputs=3
  Bus Creator2 : BusCreator  Inputs=3
  Bus Creator3 : BusCreator  Inputs=4
  Constant71 : Constant  Value=[0;0;0]  OutDataTypeStr=double
  Constant72 : Constant  OutDataTypeStr=double
  Constant73 : Constant  OutDataTypeStr=double
  Constant74 : Constant  OutDataTypeStr=double
  Constant{75..78} (4 alike) : Constant  Value=0  OutDataTypeStr=double
  Signal Specification : SignalSpecification  OutDataTypeStr=double  Unit=m  Dimensions=3
  Signal Specification{1..3,7} (4 alike) : SignalSpecification  OutDataTypeStr=double  Unit=m  Dimensions=1
  Signal Specification4 : SignalSpecification  OutDataTypeStr=double  Unit=s  Dimensions=1
  Signal Specification5 : SignalSpecification  OutDataTypeStr=double  Unit=rad  Dimensions=1
  Signal Specification6 : SignalSpecification  OutDataTypeStr=double  Unit=rad  Dimensions=1
  busGNSS : Outport
  wires:
  Bus Creator1/1 -> busGNSS/1
  Signal Specification4/1 -> Bus Creator3/1  "timestamp"
  Constant75/1 -> Signal Specification4/1
  Signal Specification/1 -> Bus Creator/1  "positionBodyToSensor"
  Signal Specification2/1 -> Bus Creator2/2  "east"
  Constant74/1 -> Signal Specification3/1
  Bus Creator/1 -> Bus Creator1/1  "alignment"
  Signal Specification3/1 -> Bus Creator2/3  "down"
  Bus Creator3/1 -> Bus Creator1/3  "measurement"
  Bus Creator2/1 -> Bus Creator1/2  "standardDeviation"
  Signal Specification5/1 -> Bus Creator3/2  "latitude"
  Constant78/1 -> Signal Specification7/1
  Signal Specification7/1 -> Bus Creator3/4  "altitude"
  Constant73/1 -> Signal Specification2/1
  Constant71/1 -> Signal Specification/1
  Constant76/1 -> Signal Specification5/1
  Constant77/1 -> Signal Specification6/1
  Signal Specification1/1 -> Bus Creator2/1  "north"
  Constant72/1 -> Signal Specification1/1
  Signal Specification6/1 -> Bus Creator3/3  "longitude"

== system GenericINSLibrary/Empty Bus Sensor Fusion No Bias Estimation/GNSS3 ==
  Bus Creator : BusCreator  Inputs=1
  Bus Creator1 : BusCreator  Inputs=3
  Bus Creator2 : BusCreator  Inputs=3
  Bus Creator3 : BusCreator  Inputs=4
  Constant71 : Constant  Value=[0;0;0]  OutDataTypeStr=double
  Constant72 : Constant  OutDataTypeStr=double
  Constant73 : Constant  OutDataTypeStr=double
  Constant74 : Constant  OutDataTypeStr=double
  Constant{75..78} (4 alike) : Constant  Value=0  OutDataTypeStr=double
  Signal Specification : SignalSpecification  OutDataTypeStr=double  Unit=m  Dimensions=3
  Signal Specification{1..3,7} (4 alike) : SignalSpecification  OutDataTypeStr=double  Unit=m  Dimensions=1
  Signal Specification4 : SignalSpecification  OutDataTypeStr=double  Unit=s  Dimensions=1
  Signal Specification5 : SignalSpecification  OutDataTypeStr=double  Unit=rad  Dimensions=1
  Signal Specification6 : SignalSpecification  OutDataTypeStr=double  Unit=rad  Dimensions=1
  busGNSS : Outport
  wires:
  Signal Specification6/1 -> Bus Creator3/3  "longitude"
  Constant72/1 -> Signal Specification1/1
  Signal Specification1/1 -> Bus Creator2/1  "north"
  Constant77/1 -> Signal Specification6/1
  Constant76/1 -> Signal Specification5/1
  Constant71/1 -> Signal Specification/1
  Constant73/1 -> Signal Specification2/1
  Signal Specification7/1 -> Bus Creator3/4  "altitude"
  Constant78/1 -> Signal Specification7/1
  Signal Specification5/1 -> Bus Creator3/2  "latitude"
  Bus Creator2/1 -> Bus Creator1/2  "standardDeviation"
  Bus Creator3/1 -> Bus Creator1/3  "measurement"
  Signal Specification3/1 -> Bus Creator2/3  "down"
  Bus Creator/1 -> Bus Creator1/1  "alignment"
  Constant74/1 -> Signal Specification3/1
  Signal Specification2/1 -> Bus Creator2/2  "east"
  Signal Specification/1 -> Bus Creator/1  "positionBodyToSensor"
  Constant75/1 -> Signal Specification4/1
  Signal Specification4/1 -> Bus Creator3/1  "timestamp"
  Bus Creator1/1 -> busGNSS/1

== system GenericINSLibrary/Empty Bus Sensor Fusion No Bias Estimation/GNSS4 ==
  Bus Creator : BusCreator  Inputs=1
  Bus Creator1 : BusCreator  Inputs=3
  Bus Creator2 : BusCreator  Inputs=3
  Bus Creator3 : BusCreator  Inputs=4
  Constant71 : Constant  Value=[0;0;0]  OutDataTypeStr=double
  Constant72 : Constant  OutDataTypeStr=double
  Constant73 : Constant  OutDataTypeStr=double
  Constant74 : Constant  OutDataTypeStr=double
  Constant{75..78} (4 alike) : Constant  Value=0  OutDataTypeStr=double
  Signal Specification : SignalSpecification  OutDataTypeStr=double  Unit=m  Dimensions=3
  Signal Specification{1..3,7} (4 alike) : SignalSpecification  OutDataTypeStr=double  Unit=m  Dimensions=1
  Signal Specification4 : SignalSpecification  OutDataTypeStr=double  Unit=s  Dimensions=1
  Signal Specification5 : SignalSpecification  OutDataTypeStr=double  Unit=rad  Dimensions=1
  Signal Specification6 : SignalSpecification  OutDataTypeStr=double  Unit=rad  Dimensions=1
  busGNSS : Outport
  wires:
  Bus Creator1/1 -> busGNSS/1
  Signal Specification4/1 -> Bus Creator3/1  "timestamp"
  Constant75/1 -> Signal Specification4/1
  Signal Specification/1 -> Bus Creator/1  "positionBodyToSensor"
  Signal Specification2/1 -> Bus Creator2/2  "east"
  Constant74/1 -> Signal Specification3/1
  Bus Creator/1 -> Bus Creator1/1  "alignment"
  Signal Specification3/1 -> Bus Creator2/3  "down"
  Bus Creator3/1 -> Bus Creator1/3  "measurement"
  Bus Creator2/1 -> Bus Creator1/2  "standardDeviation"
  Signal Specification5/1 -> Bus Creator3/2  "latitude"
  Constant78/1 -> Signal Specification7/1
  Signal Specification7/1 -> Bus Creator3/4  "altitude"
  Constant73/1 -> Signal Specification2/1
  Constant71/1 -> Signal Specification/1
  Constant76/1 -> Signal Specification5/1
  Constant77/1 -> Signal Specification6/1
  Signal Specification1/1 -> Bus Creator2/1  "north"
  Constant72/1 -> Signal Specification1/1
  Signal Specification6/1 -> Bus Creator3/3  "longitude"

== system GenericINSLibrary/Empty Bus Sensor Fusion No Bias Estimation/GNSS5 ==
  Bus Creator : BusCreator  Inputs=1
  Bus Creator1 : BusCreator  Inputs=3
  Bus Creator2 : BusCreator  Inputs=3
  Bus Creator3 : BusCreator  Inputs=4
  Constant71 : Constant  Value=[0;0;0]  OutDataTypeStr=double
  Constant72 : Constant  OutDataTypeStr=double
  Constant73 : Constant  OutDataTypeStr=double
  Constant74 : Constant  OutDataTypeStr=double
  Constant{75..78} (4 alike) : Constant  Value=0  OutDataTypeStr=double
  Signal Specification : SignalSpecification  OutDataTypeStr=double  Unit=m  Dimensions=3
  Signal Specification{1..3,7} (4 alike) : SignalSpecification  OutDataTypeStr=double  Unit=m  Dimensions=1
  Signal Specification4 : SignalSpecification  OutDataTypeStr=double  Unit=s  Dimensions=1
  Signal Specification5 : SignalSpecification  OutDataTypeStr=double  Unit=rad  Dimensions=1
  Signal Specification6 : SignalSpecification  OutDataTypeStr=double  Unit=rad  Dimensions=1
  busGNSS : Outport
  wires:
  Signal Specification6/1 -> Bus Creator3/3  "longitude"
  Constant72/1 -> Signal Specification1/1
  Signal Specification1/1 -> Bus Creator2/1  "north"
  Constant77/1 -> Signal Specification6/1
  Constant76/1 -> Signal Specification5/1
  Constant71/1 -> Signal Specification/1
  Constant73/1 -> Signal Specification2/1
  Signal Specification7/1 -> Bus Creator3/4  "altitude"
  Constant78/1 -> Signal Specification7/1
  Signal Specification5/1 -> Bus Creator3/2  "latitude"
  Bus Creator2/1 -> Bus Creator1/2  "standardDeviation"
  Bus Creator3/1 -> Bus Creator1/3  "measurement"
  Signal Specification3/1 -> Bus Creator2/3  "down"
  Bus Creator/1 -> Bus Creator1/1  "alignment"
  Constant74/1 -> Signal Specification3/1
  Signal Specification2/1 -> Bus Creator2/2  "east"
  Signal Specification/1 -> Bus Creator/1  "positionBodyToSensor"
  Constant75/1 -> Signal Specification4/1
  Signal Specification4/1 -> Bus Creator3/1  "timestamp"
  Bus Creator1/1 -> busGNSS/1
